simulink model "hireAdnFireV2"  (R2016b)
settings: Solver=ode4  StartTime=0.0  StopTime=100.0  FixedStep=0.01  RelTol=1e-3
settings Model: Creator=Thomas  LastModifiedBy=Thomas

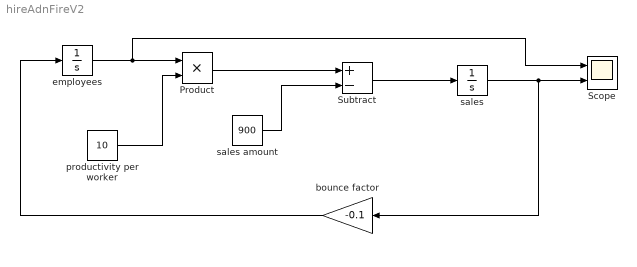
== system hireAdnFireV2 ==
  Product : Product
  Scope : Scope  NumInputPorts=2
  Subtract : Sum  Inputs=+-
  bounce factor : Gain  Gain=-0.1
  employees : Integrator  InitialCondition=50
  productivity per worker : Constant  Value=10
  sales : Integrator  InitialCondition=100
  sales amount : Constant  Value=900
  wires:
  productivity per worker/1 -> Product/2
  employees/1 -> Scope/1, Product/1
  Product/1 -> Subtract/1
  sales/1 -> bounce factor/1, Scope/2
  sales amount/1 -> Subtract/2
  Subtract/1 -> sales/1
  bounce factor/1 -> employees/1
